simulink model "Copy_of_SEIRS_PRBS"  (R2024a)
settings: Solver=VariableStepAuto  StartTime=0.0  StopTime=T  RelTol=1e-3
model workspace (MAT data in the model file):
  x = [0.0844291205376 0.0972801431163 0.171504041231 0.000911075297271]
values from neighbouring files (symbols this model uses):
  Rango_PRBS = [0.3 0.7]    [datos_2.mat]
undefined symbols (not defined in the file or in its folder): Control_U, idinput, var_init
libraries: simulink x1
settings Model: Creator=carlo  LastModifiedBy=luism
settings DataIOCC: SaveOutput=off
settings RTWCC: GPUComputeCapability=3.5

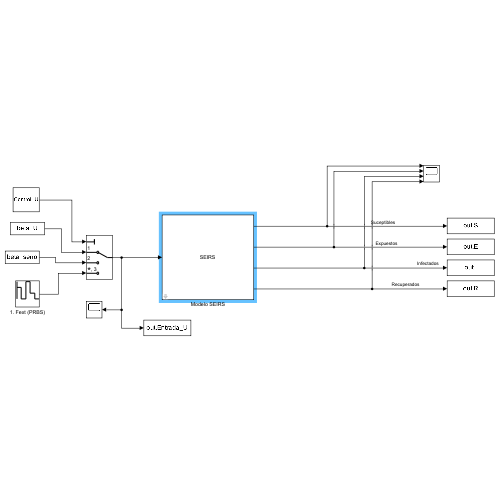
[thumbnail: Simulink's stored preview of the top-level diagram]
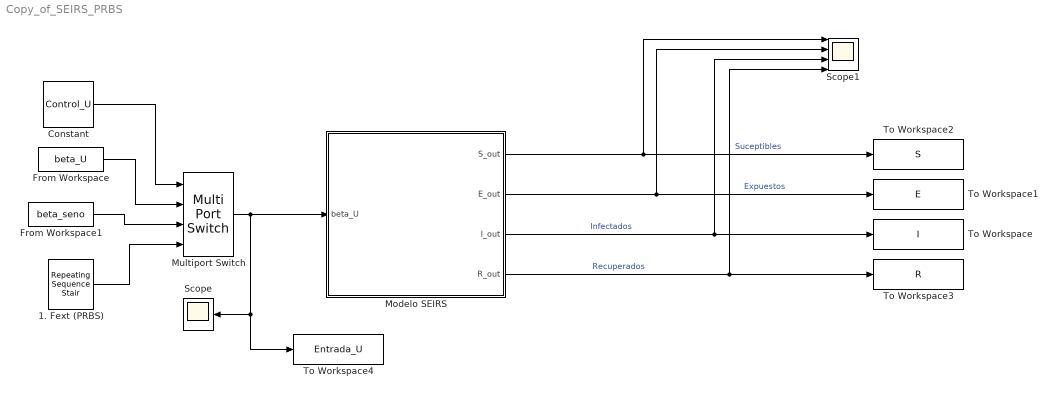
== system Copy_of_SEIRS_PRBS ==
  1. Fext (PRBS) : simulink/Sources/Repeating Sequence Stair  OutValues=idinput([2001, 1, 1], 'PRBS', [0, 1/1], [Rango_PRBS(1),Rango_PRBS(2)])  tsamp=10  OutMin=[]  OutMax=[]  OutDataTypeStr=double  OutputDataTypeScalingMode=double  OutDataType=fixdt(0,8)  ConRadixGroup=Best Precision: Vector-wise  OutScaling=2^-12
  Constant : Constant  Value=Control_U
  From Workspace : FromWorkspace  VariableName=beta_U
  From Workspace1 : FromWorkspace  VariableName=beta_seno
  Modelo SEIRS : Subsystem  mask{B=var_init(1), d=var_init(2), alpha=var_init(3), gamma=var_init(4), beta=var_init(5), nu=var_init(6), ci=[0.1431 0.0092 0.0092 0.8384], Ruido=on}
      mask prompts: ci "[S0 E0 I0 R0]"; Ruido "Incluir ruido al sistema"
      mask Display: disp('SEIRS');
  Multiport Switch : MultiPortSwitch  SaturateOnIntegerOverflow=off  InputSameDT=off
  Scope : Scope
  Scope1 : Scope  NumInputPorts=4
  To Workspace : ToWorkspace  VariableName=I  SaveFormat=Structure With Time  SampleTime=-1
  To Workspace1 : ToWorkspace  VariableName=E  SaveFormat=Structure With Time  SampleTime=-1
  To Workspace2 : ToWorkspace  VariableName=S  SaveFormat=Structure With Time  SampleTime=-1
  To Workspace3 : ToWorkspace  VariableName=R  SaveFormat=Structure With Time  SampleTime=-1
  To Workspace4 : ToWorkspace  VariableName=Entrada_U  SaveFormat=Structure With Time  SampleTime=-1
  wires:
  1. Fext (PRBS)/1 -> Multiport Switch/4
  Multiport Switch/1 -> Modelo SEIRS/1(beta_U), Scope/1, To Workspace4/1
  From Workspace1/1 -> Multiport Switch/3
  From Workspace/1 -> Multiport Switch/2
  Constant/1 -> Multiport Switch/1
  Modelo SEIRS/2(E_out) -> To Workspace1/1, Scope1/2  "Expuestos"
  Modelo SEIRS/3("I_out ") -> To Workspace/1, Scope1/3  "Infectados"
  Modelo SEIRS/1(S_out) -> To Workspace2/1, Scope1/1  "Suceptibles"
  Modelo SEIRS/4(R_out) -> To Workspace3/1, Scope1/4  "Recuperados"

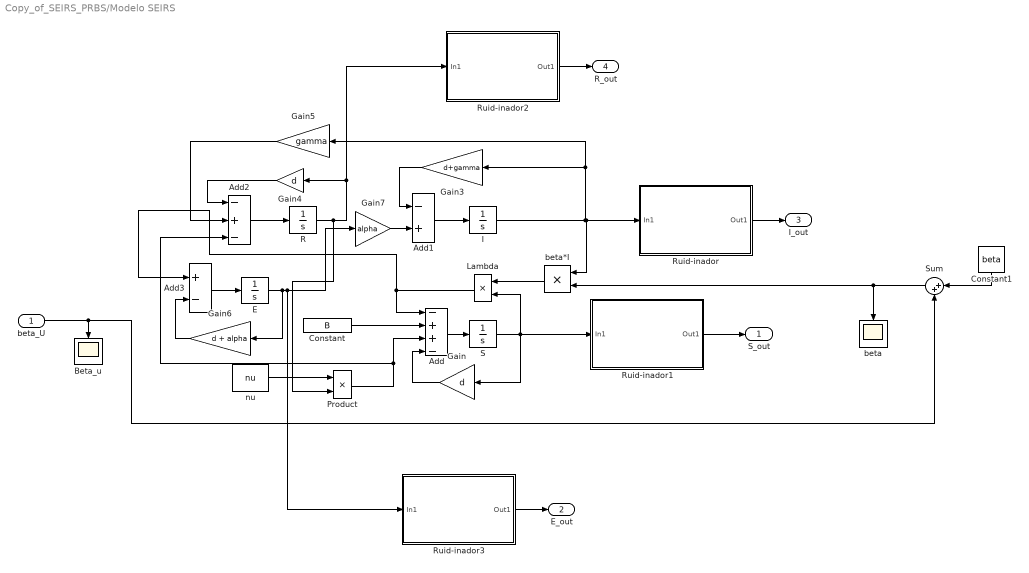
== system Copy_of_SEIRS_PRBS/Modelo SEIRS ==
  beta_U : Inport
  Add : Sum  Inputs=-++-
  Add1 : Sum  Inputs=-+
  Add2 : Sum  Inputs=-+-
  Add3 : Sum  Inputs=+-
  Beta_u : Scope
  Constant : Constant  Value=B
  Constant1 : Constant  Value=beta
  E : Integrator  InitialCondition=ci(2)  LimitOutput=on  LowerSaturationLimit=0
  Gain : Gain  Gain=d
  Gain3 : Gain  Gain=d+gamma
  Gain4 : Gain  Gain=d
  Gain5 : Gain  Gain=gamma
  Gain6 : Gain  Gain=d + alpha
  Gain7 : Gain  Gain=alpha
  I : Integrator  InitialCondition=ci(3)  LimitOutput=on  LowerSaturationLimit=0
  Lambda : Product
  Product : Product
  R : Integrator  InitialCondition=ci(4)  LimitOutput=on  LowerSaturationLimit=0
  Ruid-inador : Subsystem
      mask Display: image('ruido_inador.jpeg');
  Ruid-inador1 : Subsystem
      mask Display: image('ruido_inador.jpeg');
  Ruid-inador2 : Subsystem
      mask Display: image('ruido_inador.jpeg');
  Ruid-inador3 : Subsystem
      mask Display: image('ruido_inador.jpeg');
  S : Integrator  InitialCondition=ci(1)  LimitOutput=on  LowerSaturationLimit=0
  Sum : Sum  Inputs=|++
  beta : Scope
  beta*I : Product
  nu : Constant  Value=nu
  S_out : Outport
  E_out : Outport  Port=2
  "I_out " : Outport  Port=3
  R_out : Outport  Port=4
  wires:
  Gain/1 -> Add/4
  Gain4/1 -> Add2/1
  Constant/1 -> Add/2
  I/1 -> Ruid-inador/1(In1), beta*I/1, Gain5/1, Gain3/1
  Lambda/1 -> Add3/1, Add/1
  Add/1 -> S/1
  E/1 -> Gain7/1, Ruid-inador3/1(In1), Gain6/1
  S/1 -> Ruid-inador1/1(In1), Lambda/2, Gain/1
  Add3/1 -> E/1
  Gain3/1 -> Add1/1
  Gain5/1 -> Add2/2
  Gain6/1 -> Add3/2
  Add1/1 -> I/1
  R/1 -> Ruid-inador2/1(In1), Gain4/1, Product/2
  Add2/1 -> R/1
  Product/1 -> Add2/3, Add/3
  Gain7/1 -> Add1/2
  nu/1 -> Product/1
  beta*I/1 -> Lambda/1
  Sum/1 -> beta*I/2, beta/1
  Constant1/1 -> Sum/1
  beta_U/1 -> Sum/2, Beta_u/1
  Ruid-inador/1(Out1) -> "I_out "/1
  Ruid-inador2/1(Out1) -> R_out/1
  Ruid-inador1/1(Out1) -> S_out/1
  Ruid-inador3/1(Out1) -> E_out/1

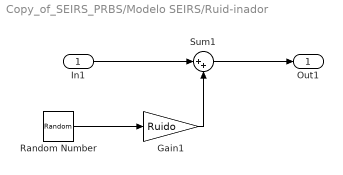
== system Copy_of_SEIRS_PRBS/Modelo SEIRS/Ruid-inador ==
  In1 : Inport
  Gain1 : Gain  Gain=Ruido
  Random Number : RandomNumber  Variance=1e-8  Seed=117  SampleTime=0.1
  Sum1 : Sum  Inputs=|++
  Out1 : Outport
  wires:
  Random Number/1 -> Gain1/1
  Gain1/1 -> Sum1/2
  In1/1 -> Sum1/1
  Sum1/1 -> Out1/1

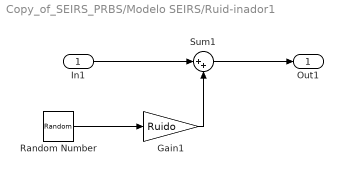
== system Copy_of_SEIRS_PRBS/Modelo SEIRS/Ruid-inador1 ==
  In1 : Inport
  Gain1 : Gain  Gain=Ruido
  Random Number : RandomNumber  Variance=1e-8  Seed=117  SampleTime=0.1
  Sum1 : Sum  Inputs=|++
  Out1 : Outport
  wires:
  Random Number/1 -> Gain1/1
  Gain1/1 -> Sum1/2
  In1/1 -> Sum1/1
  Sum1/1 -> Out1/1

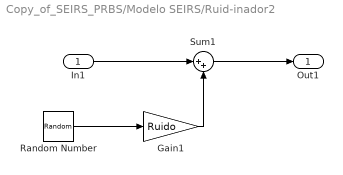
== system Copy_of_SEIRS_PRBS/Modelo SEIRS/Ruid-inador2 ==
  In1 : Inport
  Gain1 : Gain  Gain=Ruido
  Random Number : RandomNumber  Variance=1e-8  Seed=117  SampleTime=0.1
  Sum1 : Sum  Inputs=|++
  Out1 : Outport
  wires:
  Random Number/1 -> Gain1/1
  Gain1/1 -> Sum1/2
  In1/1 -> Sum1/1
  Sum1/1 -> Out1/1

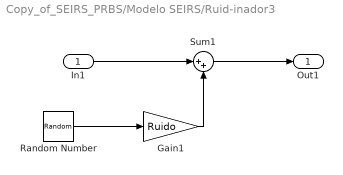
== system Copy_of_SEIRS_PRBS/Modelo SEIRS/Ruid-inador3 ==
  In1 : Inport
  Gain1 : Gain  Gain=Ruido
  Random Number : RandomNumber  Variance=1e-8  Seed=117  SampleTime=0.1
  Sum1 : Sum  Inputs=|++
  Out1 : Outport
  wires:
  Random Number/1 -> Gain1/1
  Gain1/1 -> Sum1/2
  In1/1 -> Sum1/1
  Sum1/1 -> Out1/1
